simulink library "Aerodynamics_library"  (R2022b)
settings: Solver=VariableStepAuto  StartTime=0.0  StopTime=10.0  RelTol=1e-3
undefined symbols (not defined in the file): b, c, CD0, CD_alpha, CL0, Cl_ail, CL_alpha, CL_AlphaDot, Cl_beta, CL_elev, Cl_p, CL_q, Cl_r, Cl_rud, Cm0, Cm_alpha, Cm_AlphaDot, Cm_elev, Cm_q, Cn_ail, Cn_beta, Cn_p, Cn_r, Cn_rud, CY_ail, CY_beta, CY_p, CY_r, CY_rud, S, y_cg, z_cg
settings Model: Creator=Dell  LastModifiedBy=Dell

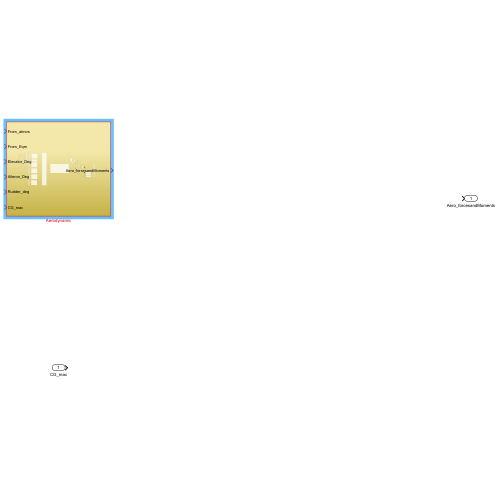
[thumbnail: Simulink's stored preview of the top-level diagram]
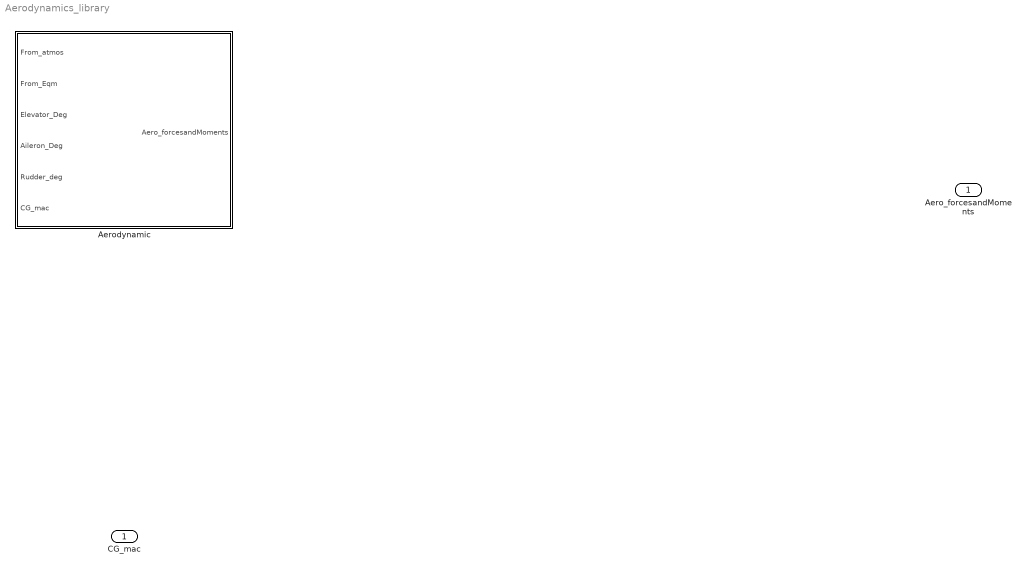
== system Aerodynamics_library ==
  CG_mac : Inport
  Aerodynamic : Subsystem
  Aero_forcesandMoments : Outport

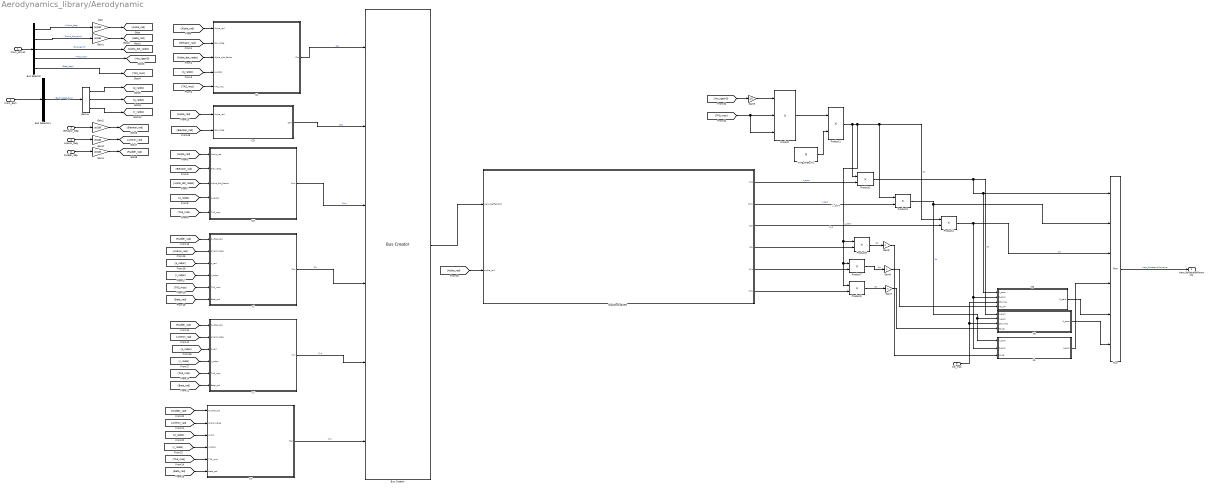
== system Aerodynamics_library/Aerodynamic ==
  note: Z_aero
  note: Cys
  From_atmos : Inport
  From_Eqm : Inport  Port=2
  Elevator_Deg : Inport  Port=3
  Aileron_Deg : Inport  Port=4
  Rudder_deg : Inport  Port=5
  CG_mac : Inport  Port=6
  Bus Creator : BusCreator  Inputs=6
  Bus Selector : BusSelector  OutputSignals=Alpha_deg,Alpha_dot_raps,Rho_kgm3,TAS_mps,Beta_deg
  Bus Selector1 : BusSelector  OutputSignals=BodyRates_Rps
  CD : Subsystem  AncestorBlock=Aerodynamics_library/CL
      settings: LibrarySourceBlock=Aerodynamics_library/CL
  CL : Subsystem
  CM : Subsystem  AncestorBlock=Aerodynamics_library/CL
      settings: LibrarySourceBlock=Aerodynamics_library/CL
  CN : Subsystem  AncestorBlock=Aerodynamics_library/Cl
      settings: LibrarySourceBlock=Aerodynamics_library/Cl
  CY : Subsystem  AncestorBlock=Aerodynamics_library/CL
      settings: LibrarySourceBlock=Aerodynamics_library/CL
  Cl : Subsystem  AncestorBlock=Aerodynamics_library/CL1
      settings: LibrarySourceBlock=Aerodynamics_library/CL1
  Demux : Demux  Outputs=3
  Gain{,1..4} (5 alike) : Gain  Gain=pi/180
  Gain5 : Gain  Gain=1/2
  Gain6 : Gain  Gain=c
  Gain7 : Gain  Gain=c
  Gain8 : Gain  Gain=c
  Lb : Subsystem
  Mb : Subsystem
  Mux : Mux  Inputs=6
  Nb : Subsystem
  Product : Product  Inputs=3
  Product{1..7} (7 alike) : Product
  Stab2body@25% : Subsystem
  wing_area_m2 : Constant  Value=S
  Aero_forcesandMoments : Outport
  wires:
  Nb/1(N_aero) -> Mux/6
  Mb/1(M_aero) -> Mux/5
  Lb/1(L_aero) -> Mux/4
  Gain8/1 -> Lb/3(Lb_cg)
  Bus Selector1/1 -> Demux/1  "<BodyRates_Rps>"
  From_Eqm/1 -> Bus Selector1/1
  Bus Selector/4 -> [rho_kgpm3]  "<TAS_mps>"
  Bus Selector/5 -> [TAS_mps]  "<Beta_deg>"
  Bus Selector/1 -> Gain/1  "<Alpha_deg>"
  From_atmos/1 -> Bus Selector/1
  CL/1(CLs) -> Bus Creator/1  "CLs"
  [r_radps] -> Cl/4(r_radps)
  [rho_kgpm3] -> Gain5/1
  [Alpha_dot_radps] -> CL/3(Alpha_dot_Radps)
  [Rudder_rad] -> Cl/1(Rudder_rad)
  [Aileron_rad] -> CN/2(aileron_Deg)
  [Elevator_rad] -> CM/2(elev_Deg)
  Product6/1 -> Gain8/1  "Qs"
  Mux/1 -> Aero_forcesandMoments/1  "Aero_forcesandMoments"
  [TAS_mps] -> Product/3, Product/2
  Product1/1 -> Product2/1, Product6/1, Product5/1, Product7/1, Product3/1, Product4/1  "Qs"
  [TAS_mps] -> CY/5(TAS_mps)
  [Aileron_rad] -> CY/2(aileron_Deg)
  [p_radps] -> CN/3(p_rad)
  [Alpha_rad] -> CM/1(Alpha_rad)
  Stab2body@25%/5(Cyb) -> Product7/2
  Bus Selector/3 -> [Alpha_dot_radps]  "<Rho_kgm3>"
  Gain/1 -> [Alpha_rad]
  Gain5/1 -> Product/1
  Rudder_deg/1 -> Gain4/1
  Product2/1 -> Mux/1, Mb/1(X_aero), Nb/1(X_aero)  "Qs"
  [TAS_mps] -> Cl/5(TAS_mps)
  [q_radps] -> CM/4(q_radps)
  [TAS_mps] -> CL/5(TAS_mps)
  [Alpha_rad] -> CL/1(Alpha_rad)
  Product4/1 -> Mux/3, Mb/2(Z_aero), Lb/2(Z_aero)  "Qs"
  Bus Creator/1 -> Stab2body@25%/1(aero-coeffecients)
  Gain3/1 -> [Aileron_rad]
  Gain1/1 -> [Beta_rad]
  Stab2body@25%/3(Czb) -> Product4/2  "Z_aero"
  [Beta_rad] -> Cl/6(Beta_rad)
  CM/1(Cms) -> Bus Creator/3  "Cms"
  [TAS_mps] -> CM/5(TAS_mps)
  Gain4/1 -> [Rudder_rad]
  Product3/1 -> Mux/2, Nb/2(Y_aero), Lb/1(Y_aero)  "Qs"
  Demux/3 -> [r_radps]
  Bus Selector/2 -> Gain1/1  "<Alpha_dot_raps>"
  [Rudder_rad] -> CY/1(Rudder_rad)
  Elevator_Deg/1 -> Gain2/1
  CD/1(CDs) -> Bus Creator/2  "CDs"
  [TAS_mps] -> CN/5(TAS_mps)
  [Elevator_rad] -> CD/2(elev_Deg)
  [p_radps] -> CY/3(p_rad)
  Stab2body@25%/6(Cnb) -> Product5/2
  Gain2/1 -> [Elevator_rad]
  Demux/1 -> [p_radps]
  Cl/1(CLs) -> Bus Creator/4  "Cls"
  Aileron_Deg/1 -> Gain3/1
  [p_radps] -> Cl/3(p_rad)
  Demux/2 -> [q_radps]
  Gain6/1 -> Mb/4(Mb_NM)
  CG_mac/1 -> Nb/3(CG_mac1), Mb/3(CG_mac)
  [Rudder_rad] -> CN/1(Rudder_rad)
  CY/1(CYs) -> Bus Creator/5  "Cys"
  [Beta_rad] -> CY/6(Beta_rad)
  [Aileron_rad] -> Cl/2(aileron_Deg)
  [r_radps] -> CY/4(r_radps)
  [q_radps] -> CL/4(q_radps)
  [Alpha_dot_radps] -> CM/3(Alpha_dot_Radps)
  [Elevator_rad] -> CL/2(elev_Deg)
  [Alpha_rad] -> CD/1(Alpha_rad)
  [Beta_rad] -> CN/6(Beta_rad)
  [r_radps] -> CN/4(r_radps)
  Stab2body@25%/2(Cmb) -> Product3/2  "Y_aero"
  Stab2body@25%/1(Cxb) -> Product2/2  "X_aero"
  Stab2body@25%/4(Clb) -> Product6/2
  CN/1(CNs) -> Bus Creator/6  "Cns"
  wing_area_m2/1 -> Product1/2
  Product7/1 -> Gain6/1  "Qs"
  Product5/1 -> Gain7/1  "Qs"
  Product/1 -> Product1/1
  Gain7/1 -> Nb/4(Nb_cg)
  [Alpha_rad] -> Stab2body@25%/2(alpha_rad)

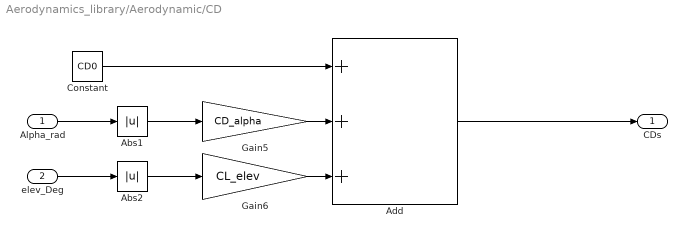
== system Aerodynamics_library/Aerodynamic/CD ==
  Alpha_rad : Inport
  elev_Deg : Inport  Port=2
  Abs1 : Abs  SaturateOnIntegerOverflow=off
  Abs2 : Abs  SaturateOnIntegerOverflow=off
  Add : Sum  Inputs=+++
  Constant : Constant  Value=CD0
  Gain5 : Gain  Gain=CD_alpha
  Gain6 : Gain  Gain=CL_elev
  CDs : Outport
  wires:
  elev_Deg/1 -> Abs2/1
  Alpha_rad/1 -> Abs1/1
  Gain5/1 -> Add/2
  Add/1 -> CDs/1
  Gain6/1 -> Add/3
  Constant/1 -> Add/1
  Abs1/1 -> Gain5/1
  Abs2/1 -> Gain6/1

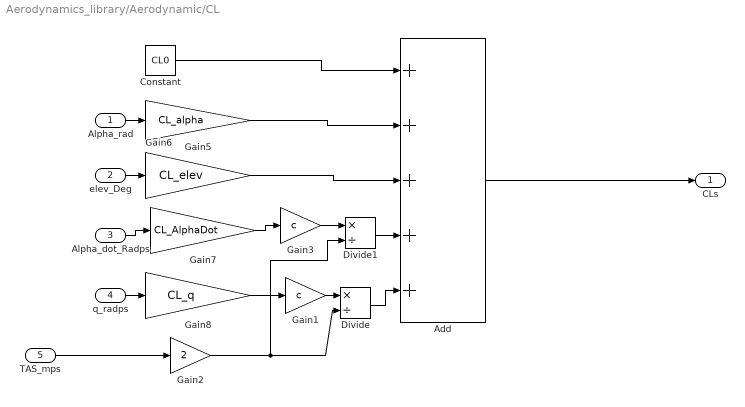
== system Aerodynamics_library/Aerodynamic/CL ==
  Alpha_rad : Inport
  elev_Deg : Inport  Port=2
  Alpha_dot_Radps : Inport  Port=3
  q_radps : Inport  Port=4
  TAS_mps : Inport  Port=5
  Add : Sum  Inputs=+++++
  Constant : Constant  Value=CL0
  Divide : Product  Inputs=*/
  Divide1 : Product  Inputs=*/
  Gain1 : Gain  Gain=c
  Gain2 : Gain  Gain=2
  Gain3 : Gain  Gain=c
  Gain5 : Gain  Gain=CL_alpha
  Gain6 : Gain  Gain=CL_elev
  Gain7 : Gain  Gain=CL_AlphaDot
  Gain8 : Gain  Gain=CL_q
  CLs : Outport
  wires:
  q_radps/1 -> Gain8/1
  elev_Deg/1 -> Gain6/1
  Alpha_dot_Radps/1 -> Gain7/1
  Alpha_rad/1 -> Gain5/1
  Gain5/1 -> Add/2
  Constant/1 -> Add/1
  Gain6/1 -> Add/3
  Add/1 -> CLs/1
  Gain8/1 -> Gain1/1
  TAS_mps/1 -> Gain2/1
  Divide/1 -> Add/5
  Gain1/1 -> Divide/1
  Gain2/1 -> Divide/2, Divide1/2
  Divide1/1 -> Add/4
  Gain3/1 -> Divide1/1
  Gain7/1 -> Gain3/1

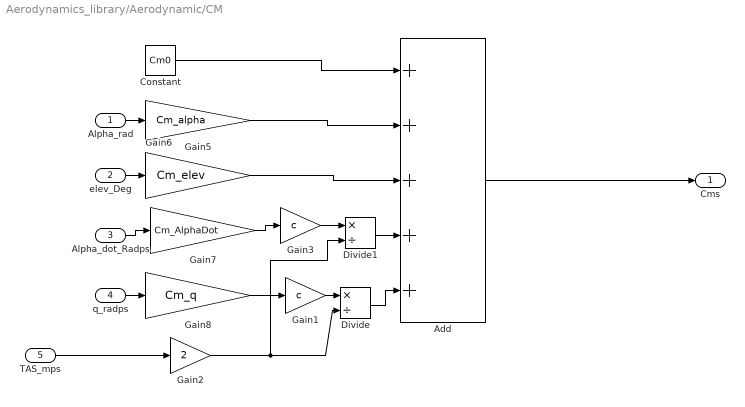
== system Aerodynamics_library/Aerodynamic/CM ==
  Alpha_rad : Inport
  elev_Deg : Inport  Port=2
  Alpha_dot_Radps : Inport  Port=3
  q_radps : Inport  Port=4
  TAS_mps : Inport  Port=5
  Add : Sum  Inputs=+++++
  Constant : Constant  Value=Cm0
  Divide : Product  Inputs=*/
  Divide1 : Product  Inputs=*/
  Gain1 : Gain  Gain=c
  Gain2 : Gain  Gain=2
  Gain3 : Gain  Gain=c
  Gain5 : Gain  Gain=Cm_alpha
  Gain6 : Gain  Gain=Cm_elev
  Gain7 : Gain  Gain=Cm_AlphaDot
  Gain8 : Gain  Gain=Cm_q
  Cms : Outport
  wires:
  q_radps/1 -> Gain8/1
  elev_Deg/1 -> Gain6/1
  Alpha_dot_Radps/1 -> Gain7/1
  Alpha_rad/1 -> Gain5/1
  Gain5/1 -> Add/2
  Constant/1 -> Add/1
  Gain6/1 -> Add/3
  Add/1 -> Cms/1
  Gain8/1 -> Gain1/1
  TAS_mps/1 -> Gain2/1
  Divide/1 -> Add/5
  Gain1/1 -> Divide/1
  Gain2/1 -> Divide/2, Divide1/2
  Divide1/1 -> Add/4
  Gain3/1 -> Divide1/1
  Gain7/1 -> Gain3/1

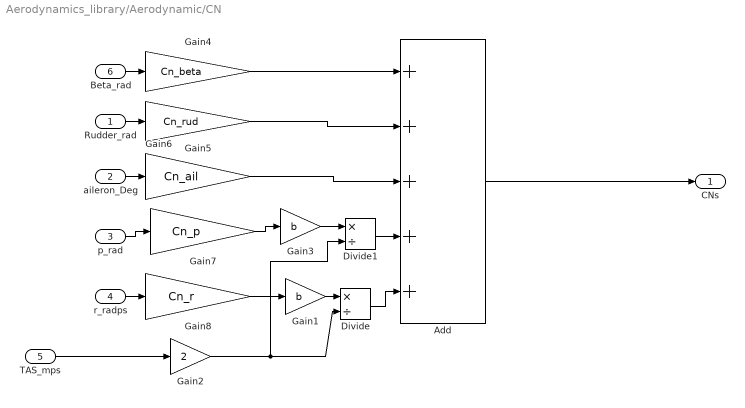
== system Aerodynamics_library/Aerodynamic/CN ==
  Rudder_rad : Inport
  aileron_Deg : Inport  Port=2
  p_rad : Inport  Port=3
  r_radps : Inport  Port=4
  TAS_mps : Inport  Port=5
  Beta_rad : Inport  Port=6
  Add : Sum  Inputs=+++++
  Divide : Product  Inputs=*/
  Divide1 : Product  Inputs=*/
  Gain1 : Gain  Gain=b
  Gain2 : Gain  Gain=2
  Gain3 : Gain  Gain=b
  Gain4 : Gain  Gain=Cn_beta
  Gain5 : Gain  Gain=Cn_rud
  Gain6 : Gain  Gain=Cn_ail
  Gain7 : Gain  Gain=Cn_p
  Gain8 : Gain  Gain=Cn_r
  CNs : Outport
  wires:
  r_radps/1 -> Gain8/1
  aileron_Deg/1 -> Gain6/1
  p_rad/1 -> Gain7/1
  Rudder_rad/1 -> Gain5/1
  Gain5/1 -> Add/2
  Gain6/1 -> Add/3
  Add/1 -> CNs/1
  Gain8/1 -> Gain1/1
  TAS_mps/1 -> Gain2/1
  Divide/1 -> Add/5
  Gain1/1 -> Divide/1
  Gain2/1 -> Divide/2, Divide1/2
  Divide1/1 -> Add/4
  Gain3/1 -> Divide1/1
  Gain7/1 -> Gain3/1
  Gain4/1 -> Add/1
  Beta_rad/1 -> Gain4/1

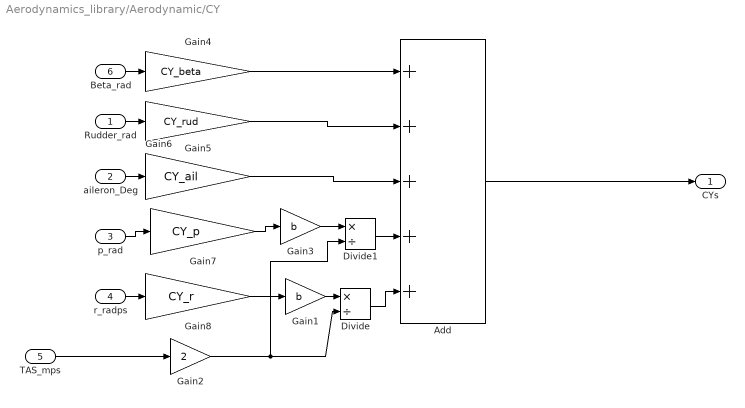
== system Aerodynamics_library/Aerodynamic/CY ==
  Rudder_rad : Inport
  aileron_Deg : Inport  Port=2
  p_rad : Inport  Port=3
  r_radps : Inport  Port=4
  TAS_mps : Inport  Port=5
  Beta_rad : Inport  Port=6
  Add : Sum  Inputs=+++++
  Divide : Product  Inputs=*/
  Divide1 : Product  Inputs=*/
  Gain1 : Gain  Gain=b
  Gain2 : Gain  Gain=2
  Gain3 : Gain  Gain=b
  Gain4 : Gain  Gain=CY_beta
  Gain5 : Gain  Gain=CY_rud
  Gain6 : Gain  Gain=CY_ail
  Gain7 : Gain  Gain=CY_p
  Gain8 : Gain  Gain=CY_r
  CYs : Outport
  wires:
  r_radps/1 -> Gain8/1
  aileron_Deg/1 -> Gain6/1
  p_rad/1 -> Gain7/1
  Rudder_rad/1 -> Gain5/1
  Gain5/1 -> Add/2
  Gain6/1 -> Add/3
  Add/1 -> CYs/1
  Gain8/1 -> Gain1/1
  TAS_mps/1 -> Gain2/1
  Divide/1 -> Add/5
  Gain1/1 -> Divide/1
  Gain2/1 -> Divide/2, Divide1/2
  Divide1/1 -> Add/4
  Gain3/1 -> Divide1/1
  Gain7/1 -> Gain3/1
  Gain4/1 -> Add/1
  Beta_rad/1 -> Gain4/1

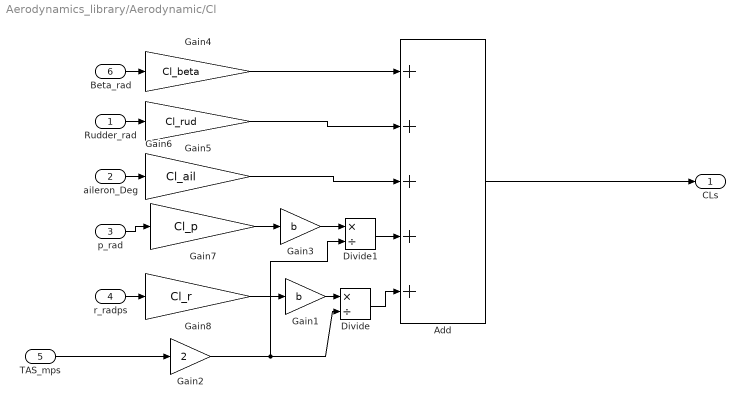
== system Aerodynamics_library/Aerodynamic/Cl ==
  Rudder_rad : Inport
  aileron_Deg : Inport  Port=2
  p_rad : Inport  Port=3
  r_radps : Inport  Port=4
  TAS_mps : Inport  Port=5
  Beta_rad : Inport  Port=6
  Add : Sum  Inputs=+++++
  Divide : Product  Inputs=*/
  Divide1 : Product  Inputs=*/
  Gain1 : Gain  Gain=b
  Gain2 : Gain  Gain=2
  Gain3 : Gain  Gain=b
  Gain4 : Gain  Gain=Cl_beta
  Gain5 : Gain  Gain=Cl_rud
  Gain6 : Gain  Gain=Cl_ail
  Gain7 : Gain  Gain=Cl_p
  Gain8 : Gain  Gain=Cl_r
  CLs : Outport
  wires:
  r_radps/1 -> Gain8/1
  aileron_Deg/1 -> Gain6/1
  p_rad/1 -> Gain7/1
  Rudder_rad/1 -> Gain5/1
  Gain5/1 -> Add/2
  Gain6/1 -> Add/3
  Add/1 -> CLs/1
  Gain8/1 -> Gain1/1
  TAS_mps/1 -> Gain2/1
  Divide/1 -> Add/5
  Gain1/1 -> Divide/1
  Gain2/1 -> Divide/2, Divide1/2
  Divide1/1 -> Add/4
  Gain3/1 -> Divide1/1
  Gain7/1 -> Gain3/1
  Gain4/1 -> Add/1
  Beta_rad/1 -> Gain4/1

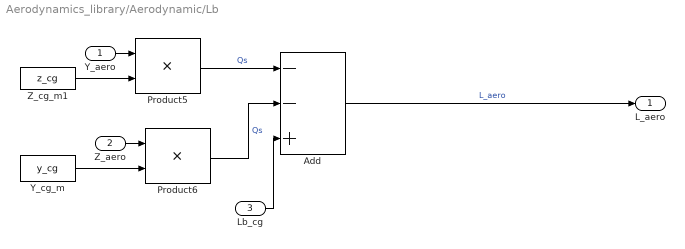
== system Aerodynamics_library/Aerodynamic/Lb ==
  Y_aero : Inport
  Z_aero : Inport  Port=2
  Lb_cg : Inport  Port=3
  Add : Sum  Inputs=--+
  Product5 : Product
  Product6 : Product
  Y_cg_m : Constant  Value=y_cg
  Z_cg_m1 : Constant  Value=z_cg
  L_aero : Outport
  wires:
  Product5/1 -> Add/1  "Qs"
  Z_cg_m1/1 -> Product5/2
  Y_aero/1 -> Product5/1
  Lb_cg/1 -> Add/3
  Add/1 -> L_aero/1  "L_aero"
  Product6/1 -> Add/2  "Qs"
  Y_cg_m/1 -> Product6/2
  Z_aero/1 -> Product6/1

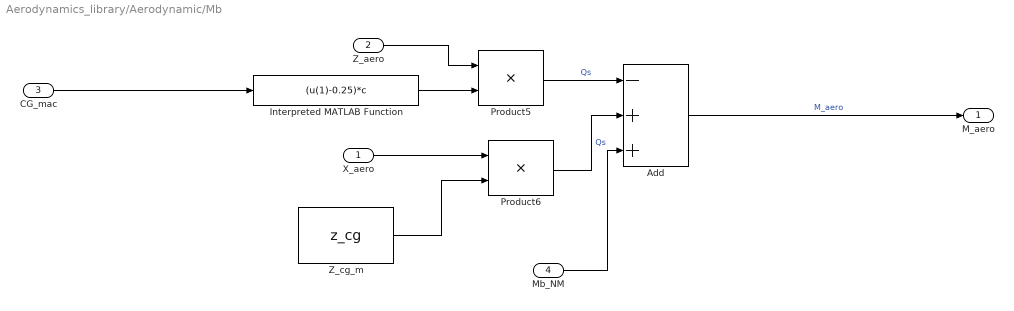
== system Aerodynamics_library/Aerodynamic/Mb ==
  X_aero : Inport
  Z_aero : Inport  Port=2
  CG_mac : Inport  Port=3
  Mb_NM : Inport  Port=4
  Add : Sum  Inputs=-++
  Interpreted MATLAB Function : MATLABFcn  MATLABFcn=(u(1)-0.25)*c  OutputDimensions=1
  Product5 : Product
  Product6 : Product
  Z_cg_m : Constant  Value=z_cg
  M_aero : Outport
  wires:
  Product5/1 -> Add/1  "Qs"
  Interpreted MATLAB Function/1 -> Product5/2
  CG_mac/1 -> Interpreted MATLAB Function/1
  Z_cg_m/1 -> Product6/2
  Mb_NM/1 -> Add/3
  Product6/1 -> Add/2  "Qs"
  Add/1 -> M_aero/1  "M_aero"
  X_aero/1 -> Product6/1
  Z_aero/1 -> Product5/1

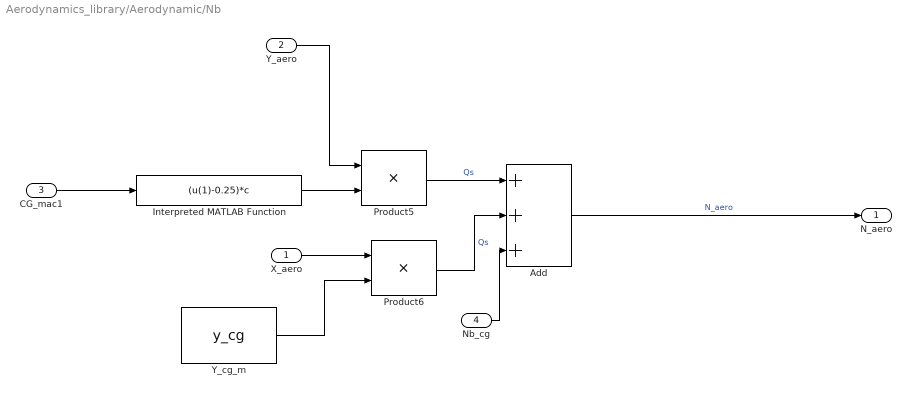
== system Aerodynamics_library/Aerodynamic/Nb ==
  X_aero : Inport
  Y_aero : Inport  Port=2
  CG_mac1 : Inport  Port=3
  Nb_cg : Inport  Port=4
  Add : Sum  Inputs=+++
  Interpreted MATLAB Function : MATLABFcn  MATLABFcn=(u(1)-0.25)*c  OutputDimensions=1
  Product5 : Product
  Product6 : Product
  Y_cg_m : Constant  Value=y_cg
  N_aero : Outport
  wires:
  X_aero/1 -> Product6/1
  Y_cg_m/1 -> Product6/2
  Product6/1 -> Add/2  "Qs"
  Add/1 -> N_aero/1  "N_aero"
  CG_mac1/1 -> Interpreted MATLAB Function/1
  Nb_cg/1 -> Add/3
  Y_aero/1 -> Product5/1
  Interpreted MATLAB Function/1 -> Product5/2
  Product5/1 -> Add/1  "Qs"

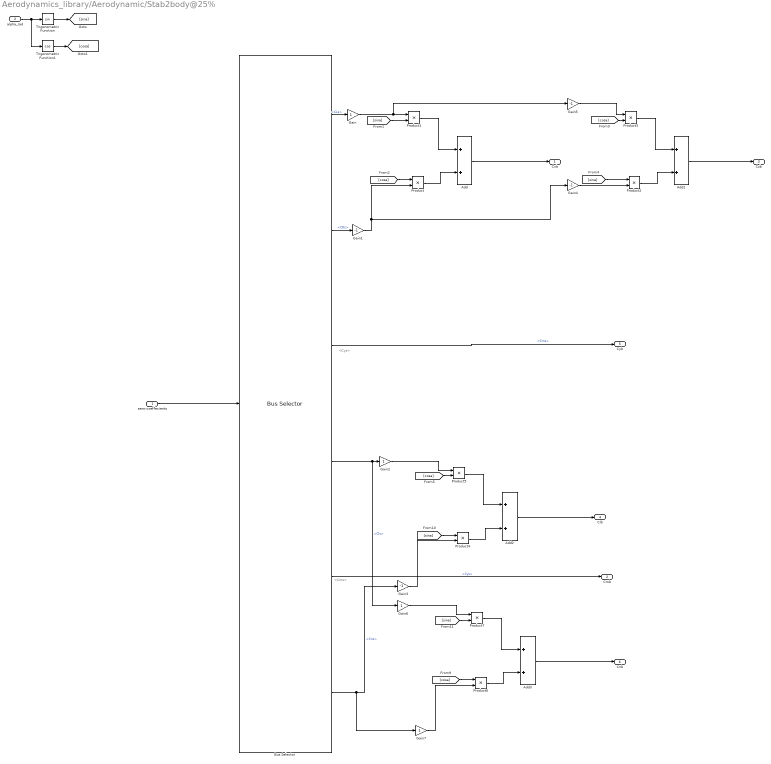
== system Aerodynamics_library/Aerodynamic/Stab2body@25% ==
  note: <Cms>
  note: <Cys>
  aero-coeffecients : Inport
  alpha_rad : Inport  Port=2
  Add{,1..3} (4 alike) : Sum
  Bus Selector : BusSelector  OutputSignals=CLs,CDs,Cms,Cls,Cys,Cns
  Gain{,2,6..7} (4 alike) : Gain
  Gain{1,3..5} (4 alike) : Gain  Gain=-1
  Product{,1..7} (8 alike) : Product
  Trigonometric Function : Trigonometry
  Trigonometric Function1 : Trigonometry  Operator=cos
  Cxb : Outport
  Cmb : Outport  Port=2
  Czb : Outport  Port=3
  Clb : Outport  Port=4
  Cyb : Outport  Port=5
  Cnb : Outport  Port=6
  wires:
  Bus Selector/5 -> Cmb/1  "<Cys>"
  Bus Selector/6 -> Gain7/1, Gain3/1  "<Cns>"
  aero-coeffecients/1 -> Bus Selector/1
  Bus Selector/2 -> Gain1/1  "<CDs>"
  Bus Selector/1 -> Gain/1  "<CLs>"
  Bus Selector/3 -> Cyb/1  "<Cms>"
  Bus Selector/4 -> Gain6/1, Gain2/1  "<Cls>"
  alpha_rad/1 -> Trigonometric Function1/1, Trigonometric Function/1
  Trigonometric Function/1 -> [sina]
  Trigonometric Function1/1 -> [cosa]
  [sina] -> Product1/2
  [cosa] -> Product/1
  Product1/1 -> Add/1
  Product/1 -> Add/2
  Add/1 -> Cxb/1
  Product2/1 -> Add1/2
  Product3/1 -> Add1/1
  Gain/1 -> Gain5/1, Product1/1
  Gain1/1 -> Gain4/1, Product/2
  [sina] -> Product2/1
  [cosa] -> Product3/2
  Add1/1 -> Czb/1
  Product4/1 -> Add2/2
  [sina] -> Product4/1
  Product5/1 -> Add2/1
  Gain3/1 -> Product4/2
  Add2/1 -> Clb/1
  Gain2/1 -> Product5/1
  [cosa] -> Product5/2
  Gain4/1 -> Product2/2
  Gain5/1 -> Product3/1
  [sina] -> Product7/2
  Add3/1 -> Cnb/1
  Gain6/1 -> Product7/1
  Gain7/1 -> Product6/2
  Product7/1 -> Add3/1
  Product6/1 -> Add3/2
  [cosa] -> Product6/1
